simulink model "impedanceControl_R2017b"  (Simulink 9.0)
settings: Solver=FixedStepDiscrete  StartTime=0.0  StopTime=Config.SIMULATION_TIME  FixedStep=Config.Ts  RelTol=1e-3  EnableMultiTasking=on
InitFcn:
  | cd(fileparts(which(bdroot)));
  | initImpedanceControl;
StopFcn:
  | cd(fileparts(which(bdroot)));
  | stopImpedanceControl;
undefined symbols (not defined in the file or in its folder): AMPLS, Config, FREQS, JTCVC_1_OR_MCC_0_SELECTOR, K0, Kc, Kd, Kfc, Kp, Kt, Kv, ROBOT_DOF, T
libraries: WBToolboxLibrary x17, simulink x1
settings Model: SuppressorTable=22 serialization::archive 11 0 6 0 0 0 1 0  Creator=daniele  LastModifiedBy=icub
settings DataIOCC: LimitDataPoints=on
settings DebuggingCC: UnderspecifiedInitializationDetection=Simplified  MergeDetectMultiDrivingBlocksExec=error  SolverPrmCheckMsg=warning  MultiTaskDSMMsg=warning  MultiTaskCondExecSysMsg=none  AllowSymbolicDim=off  StrictBusMsg=ErrorOnBusTreatedAsVector
settings GRTTargetCC: GeneratePreprocessorConditionals=Disable all

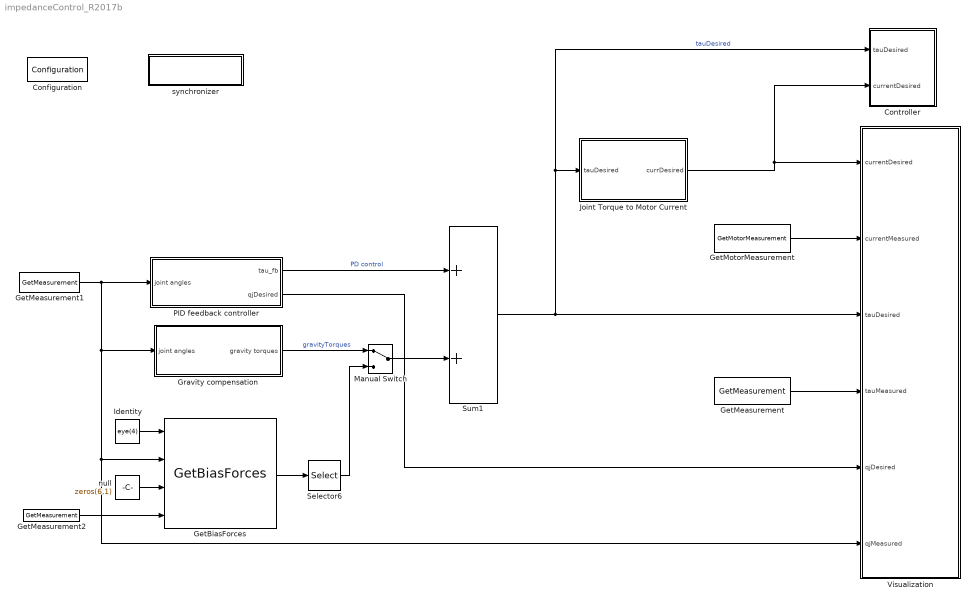
== system impedanceControl_R2017b ==
  Configuration : WBToolboxLibrary/Utilities/Configuration  ConfigSource=Workspace  ConfigObject='WBTConfigRobot'  RobotName='icubSim'  UrdfFile='model.urdf'  ControlledJoints={'l_elbow','l_shoulder_pitch','torso_roll'}  ControlBoardsNames={'left_arm','right_arm','torso'}  LocalName='WBT'  GravityVector=[0,0,-9.81]
      settings: SourceProductName=WholeBodyToolbox
  Controller : Subsystem
  GetBiasForces : WBToolboxLibrary/Model/Dynamics/GetBiasForces
      settings: SourceProductName=WholeBodyToolbox
  GetMeasurement : WBToolboxLibrary/States/GetMeasurement  measuredType=Joints Torque
      settings: SourceProductName=WholeBodyToolbox
  GetMeasurement1 : WBToolboxLibrary/States/GetMeasurement  measuredType=Joints Position
      settings: SourceProductName=WholeBodyToolbox
  GetMeasurement2 : WBToolboxLibrary/States/GetMeasurement  measuredType=Joints Velocity
      settings: SourceProductName=WholeBodyToolbox
  GetMotorMeasurement : WBToolboxLibrary/States/GetMotorMeasurement  measuredType=Motor Current
      settings: SourceProductName=WholeBodyToolbox
  Gravity compensation : Subsystem
  Identity : Constant  Value=eye(4)
  Joint Torque to Motor Current : Subsystem
  Manual Switch : ManualSwitch
  PID feedback controller : Subsystem
  Selector6 : Selector  InputPortWidth=12  IndexOptions=Index vector (dialog)  Indices=[7:12]  OutputSizes=1
  Sum1 : Sum
  Visualization : Subsystem
  null : Constant  Value=zeros(6,1)
  synchronizer : Subsystem
      mask Display: disp('SYNCHRONIZER')
  wires:
  GetMeasurement1/1 -> Visualization/6(qjMeasured), GetBiasForces/2, Gravity compensation/1(joint angles), PID feedback controller/1(joint angles)
  Gravity compensation/1(gravity torques) -> Manual Switch/1  "gravityTorques"
  Sum1/1 -> Controller/1(tauDesired), Joint Torque to Motor Current/1(tauDesired), Visualization/3(tauDesired)  "tauDesired"
  PID feedback controller/1(tau_fb) -> Sum1/1  "PD control"
  Joint Torque to Motor Current/1(currDesired) -> Visualization/1(currentDesired), Controller/2(currentDesired)
  GetMotorMeasurement/1 -> Visualization/2(currentMeasured)
  PID feedback controller/2(qjDesired) -> Visualization/5(qjDesired)
  GetMeasurement/1 -> Visualization/4(tauMeasured)
  Identity/1 -> GetBiasForces/1
  GetMeasurement2/1 -> GetBiasForces/4
  null/1 -> GetBiasForces/3
  GetBiasForces/1 -> Selector6/1
  Manual Switch/1 -> Sum1/2
  Selector6/1 -> Manual Switch/2

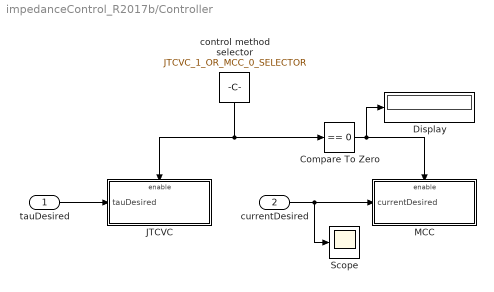
== system impedanceControl_R2017b/Controller ==
  tauDesired : Inport
  currentDesired : Inport  Port=2
  Compare To Zero : simulink/Logic and Bit Operations/Compare To Zero  relop===  OutDataTypeStr=boolean
  Display : Display
  JTCVC : Subsystem  TreatAsAtomicUnit=on
  MCC : Subsystem  TreatAsAtomicUnit=on
  Scope : Scope
  control method selector : Constant  Value=JTCVC_1_OR_MCC_0_SELECTOR
  wires:
  control method selector/1 -> JTCVC/Enable, Compare To Zero/1
  tauDesired/1 -> JTCVC/1(tauDesired)
  currentDesired/1 -> Scope/1, MCC/1(currentDesired)
  Compare To Zero/1 -> Display/1, MCC/Enable

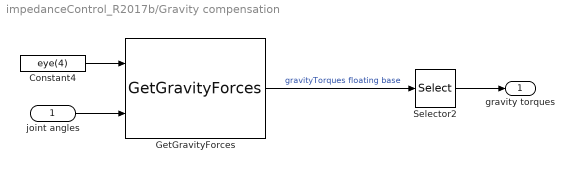
== system impedanceControl_R2017b/Gravity compensation ==
  joint angles : Inport
  Constant4 : Constant  Value=eye(4)
  GetGravityForces : WBToolboxLibrary/Model/Dynamics/GetGravityForces
      settings: SourceProductName=WholeBodyToolbox
  Selector2 : Selector  InputPortWidth=ROBOT_DOF+6  IndexOptions=Index vector (dialog)  Indices=[7:ROBOT_DOF+6]  OutputSizes=1
  gravity torques : Outport
  wires:
  Selector2/1 -> gravity torques/1
  Constant4/1 -> GetGravityForces/1
  joint angles/1 -> GetGravityForces/2
  GetGravityForces/1 -> Selector2/1  "gravityTorques floating base"

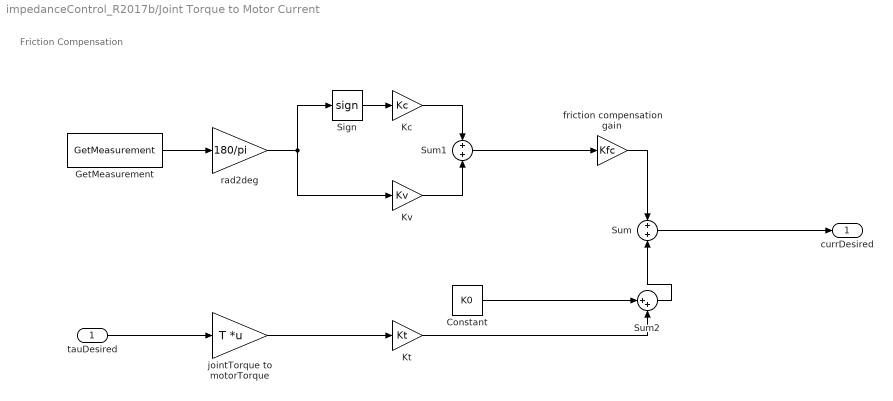
== system impedanceControl_R2017b/Joint Torque to Motor Current ==
  note: Friction Compensation
  tauDesired : Inport
  Constant : Constant  Value=K0
  GetMeasurement : WBToolboxLibrary/States/GetMeasurement  measuredType=Joints Velocity
      settings: SourceProductName=WholeBodyToolbox
  Kc : Gain  Gain=Kc
  Kt : Gain  Gain=Kt
  Kv : Gain  Gain=Kv
  Sign : Signum
  Sum : Sum
  Sum1 : Sum
  Sum2 : Sum  Inputs=|++
  friction compensation gain : Gain  Gain=Kfc
  jointTorque to motorTorque : Gain  Gain=T  Multiplication=Matrix(K*u) (u vector)
  rad2deg : Gain  Gain=180/pi
  currDesired : Outport
  wires:
  Sum/1 -> currDesired/1
  tauDesired/1 -> jointTorque to motorTorque/1
  Sign/1 -> Kc/1
  rad2deg/1 -> Kv/1, Sign/1
  Sum1/1 -> friction compensation gain/1
  friction compensation gain/1 -> Sum/1
  Kc/1 -> Sum1/1
  Kv/1 -> Sum1/2
  jointTorque to motorTorque/1 -> Kt/1
  Constant/1 -> Sum2/1
  Kt/1 -> Sum2/2
  Sum2/1 -> Sum/2
  GetMeasurement/1 -> rad2deg/1

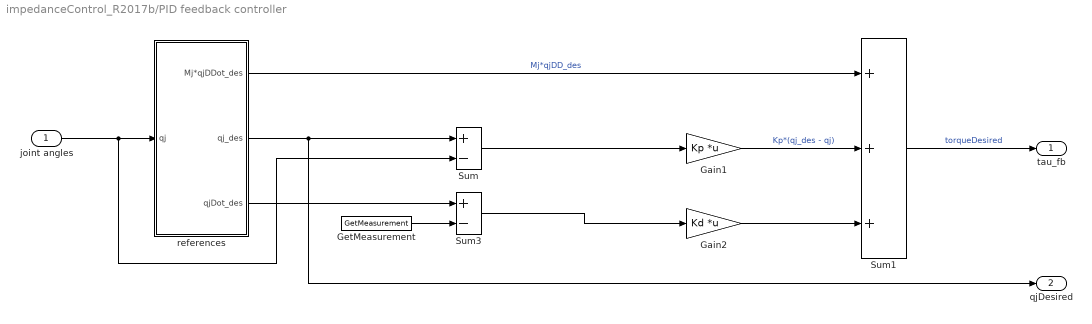
== system impedanceControl_R2017b/PID feedback controller ==
  joint angles : Inport
  Gain1 : Gain  Gain=Kp  Multiplication=Matrix(K*u)
  Gain2 : Gain  Gain=Kd  Multiplication=Matrix(K*u)
  GetMeasurement : WBToolboxLibrary/States/GetMeasurement  measuredType=Joints Velocity
      settings: SourceProductName=WholeBodyToolbox
  Sum : Sum  Inputs=+-
  Sum1 : Sum  Inputs=+++
  Sum3 : Sum  Inputs=+-
  references : Subsystem
  tau_fb : Outport
  qjDesired : Outport  Port=2
  wires:
  GetMeasurement/1 -> Sum3/2
  Sum/1 -> Gain1/1
  joint angles/1 -> Sum/2, references/1(qj)
  references/1(Mj*qjDDot_des) -> Sum1/1  "Mj*qjDD_des"
  Sum3/1 -> Gain2/1
  references/3(qjDot_des) -> Sum3/1
  Sum1/1 -> tau_fb/1  "torqueDesired"
  references/2(" qj_des") -> qjDesired/1, Sum/1
  Gain1/1 -> Sum1/2  "Kp*(qj_des - qj)"
  Gain2/1 -> Sum1/3

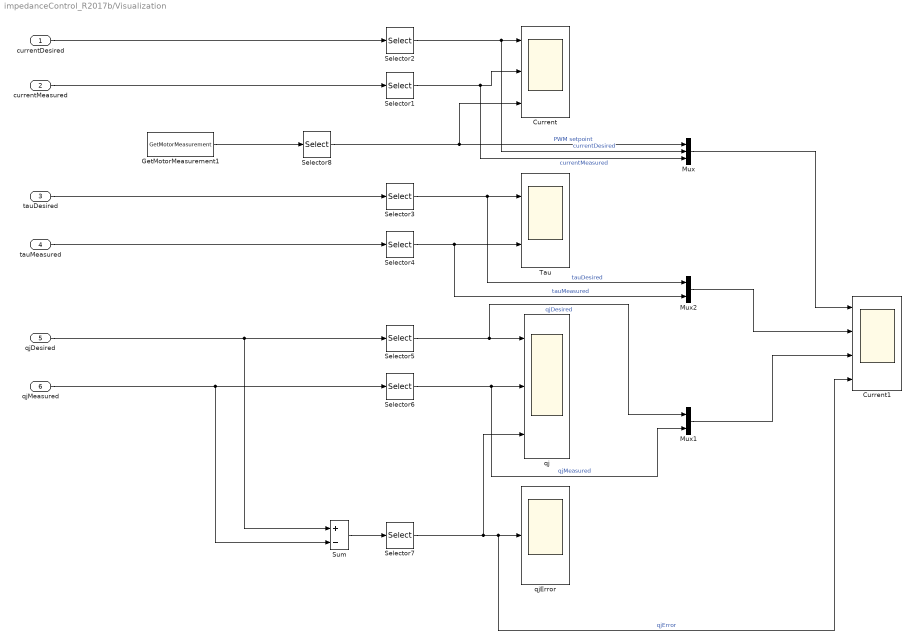
== system impedanceControl_R2017b/Visualization ==
  currentDesired : Inport
  currentMeasured : Inport  Port=2
  tauDesired : Inport  Port=3
  tauMeasured : Inport  Port=4
  qjDesired : Inport  Port=5
  qjMeasured : Inport  Port=6
  Current : Scope  NumInputPorts=3
  Current1 : Scope  NumInputPorts=4
  GetMotorMeasurement1 : WBToolboxLibrary/States/GetMotorMeasurement  measuredType=Motor PWM
      settings: SourceProductName=WholeBodyToolbox
  Mux : Mux  Inputs=3
  Mux1 : Mux  Inputs=2
  Mux2 : Mux  Inputs=2
  Selector{1..8} (8 alike) : Selector  InputPortWidth=ROBOT_DOF  IndexOptions=Index vector (dialog)  Indices=JOINTS_TO_PLOT  OutputSizes=1
  Sum : Sum  Inputs=+-
  Tau : Scope  NumInputPorts=2
  qj : Scope  NumInputPorts=3
  qjError : Scope
  wires:
  Selector5/1 -> Mux1/1, qj/1  "qjDesired"
  Selector2/1 -> Mux/2, Current/1  "currentDesired"
  Selector6/1 -> Mux1/2, qj/2  "qjMeasured"
  Selector1/1 -> Mux/3, Current/2  "currentMeasured"
  Selector3/1 -> Mux2/1, Tau/1  "tauDesired"
  Selector4/1 -> Mux2/2, Tau/2  "tauMeasured"
  currentDesired/1 -> Selector2/1
  currentMeasured/1 -> Selector1/1
  tauDesired/1 -> Selector3/1
  tauMeasured/1 -> Selector4/1
  qjDesired/1 -> Sum/1, Selector5/1
  qjMeasured/1 -> Sum/2, Selector6/1
  Sum/1 -> Selector7/1
  Selector7/1 -> qj/3, Current1/4, qjError/1  "qjError"
  Mux/1 -> Current1/1
  Mux2/1 -> Current1/2
  Mux1/1 -> Current1/3
  GetMotorMeasurement1/1 -> Selector8/1
  Selector8/1 -> Current/3, Mux/1  "PWM setpoint"

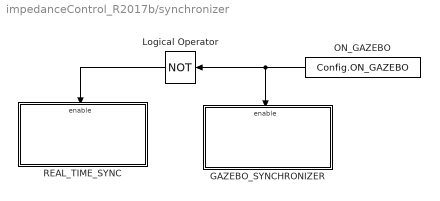
== system impedanceControl_R2017b/synchronizer ==
  GAZEBO_SYNCHRONIZER : Subsystem
  Logical Operator : Logic  Operator=NOT  AllPortsSameDT=off  OutDataTypeStr=boolean
  "ON_GAZEBO " : Constant  Value=Config.ON_GAZEBO
  REAL_TIME_SYNC : Subsystem
  wires:
  Logical Operator/1 -> REAL_TIME_SYNC/Enable
  "ON_GAZEBO "/1 -> GAZEBO_SYNCHRONIZER/Enable, Logical Operator/1

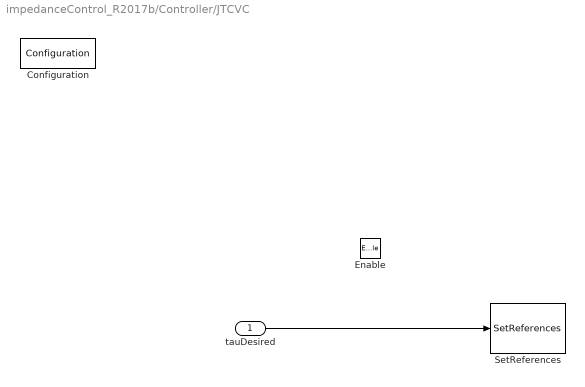
== system impedanceControl_R2017b/Controller/JTCVC ==
  tauDesired : Inport
  Enable : EnablePort
  Configuration : WBToolboxLibrary/Utilities/Configuration  ConfigSource=Workspace  ConfigObject='WBTConfigRobot2'  RobotName='icubSim'  UrdfFile='model.urdf'  ControlledJoints={'l_elbow','l_shoulder_pitch','torso_roll'}  ControlBoardsNames={'left_arm','right_arm','torso'}  LocalName='WBT'  GravityVector=[0,0,-9.81]
      settings: SourceProductName=WholeBodyToolbox
  SetReferences : WBToolboxLibrary/Actuators/SetReferences  controlType=Torque  refSpeed=10*(pi/180)  refAcceleration=1000000*(pi/180)
      settings: SourceProductName=WholeBodyToolbox
  wires:
  tauDesired/1 -> SetReferences/1

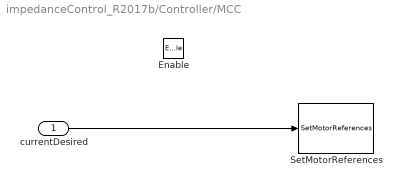
== system impedanceControl_R2017b/Controller/MCC ==
  currentDesired : Inport
  Enable : EnablePort
  SetMotorReferences : WBToolboxLibrary/Actuators/SetMotorReferences  controlType=Current
      settings: SourceProductName=WholeBodyToolbox
  wires:
  currentDesired/1 -> SetMotorReferences/1

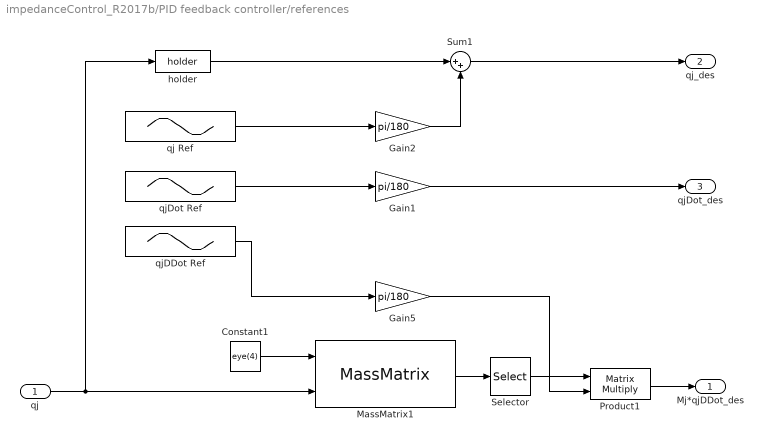
== system impedanceControl_R2017b/PID feedback controller/references ==
  qj : Inport
  Constant1 : Constant  Value=eye(4)
  Gain1 : Gain  Gain=pi/180
  Gain2 : Gain  Gain=pi/180
  Gain5 : Gain  Gain=pi/180
  MassMatrix1 : WBToolboxLibrary/Model/Dynamics/MassMatrix
      settings: SourceProductName=WholeBodyToolbox
  Product1 : Product  Multiplication=Matrix(*)
  Selector : Selector  NumberOfDimensions=2  InputPortWidth=3  IndexOptions=Index vector (dialog),Index vector (dialog)  Indices=[7:ROBOT_DOF+6],[7:ROBOT_DOF+6]  OutputSizes=1,1
  Sum1 : Sum  Inputs=|++
  holder : WBToolboxLibrary/Utilities/holder 
      settings: SourceProductName=WholeBodyToolbox
  qj Ref : Sin  Amplitude=AMPLS  Frequency=FREQS*2*pi  SampleTime=0
  qjDDot Ref : Sin  Amplitude=-AMPLS.*(FREQS*2*pi).^2  Frequency=FREQS*2*pi  SampleTime=0
  qjDot Ref : Sin  Amplitude=AMPLS.*FREQS*2*pi  Frequency=FREQS*2*pi  Phase=pi/2  SampleTime=0
  Mj*qjDDot_des : Outport
  " qj_des" : Outport  Port=2
  qjDot_des : Outport  Port=3
  wires:
  qj Ref/1 -> Gain2/1
  qjDot Ref/1 -> Gain1/1
  Product1/1 -> Mj*qjDDot_des/1
  MassMatrix1/1 -> Selector/1
  Selector/1 -> Product1/1
  qjDDot Ref/1 -> Gain5/1
  Gain5/1 -> Product1/2
  qj/1 -> holder/1, MassMatrix1/2
  holder/1 -> Sum1/1
  Constant1/1 -> MassMatrix1/1
  Gain1/1 -> qjDot_des/1
  Gain2/1 -> Sum1/2
  Sum1/1 -> " qj_des"/1

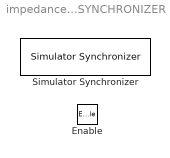
== system impedanceControl_R2017b/synchronizer/GAZEBO_SYNCHRONIZER ==
  Enable : EnablePort
  Simulator Synchronizer : WBToolboxLibrary/Utilities/Simulator Synchronizer  period=Config.Ts  serverPortName='/clock/rpc'  clientPortName='/WBT_synchronizer/rpc:o'
      settings: SourceProductName=WholeBodyToolbox

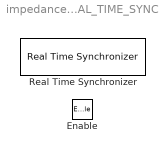
== system impedanceControl_R2017b/synchronizer/REAL_TIME_SYNC ==
  Enable : EnablePort
  Real Time Synchronizer : WBToolboxLibrary/Utilities/Real Time Synchronizer  period=Config.Ts
      settings: SourceProductName=WholeBodyToolbox
